simulink model "model_linear"  (R2022a)
settings: Solver=VariableStepAuto  StartTime=0  StopTime=100  RelTol=1e-3
values from neighbouring files (symbols this model uses):
  A = [ 0 1 0  0 ... (first row only)    [ball_and_beam_pfc.m]
  amplitude_entrada = 1    [ball_and_beam_pfc.m]
  B = [0 ... (first row only)    [ball_and_beam_pfc.m]
  bool_degrau = 1    [ball_and_beam_pfc.m]
  C = [0 0 1 0]    [ball_and_beam_pfc.m]
  k_seguimento = K_nulo(1:4)    [ball_and_beam_pfc.m]
  ki_seguimento = K_nulo(5)    [ball_and_beam_pfc.m]
  L = 0.425    [ball_and_beam_pfc.m]    (also in nonlinear_ball_and_beam.m)
libraries: vrlib x3
settings Model: Creator=Notebook_Artur  LastModifiedBy=Notebook_Artur

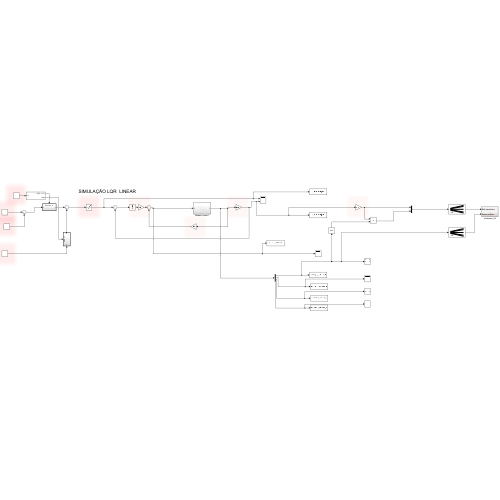
[thumbnail: Simulink's stored preview of the top-level diagram]
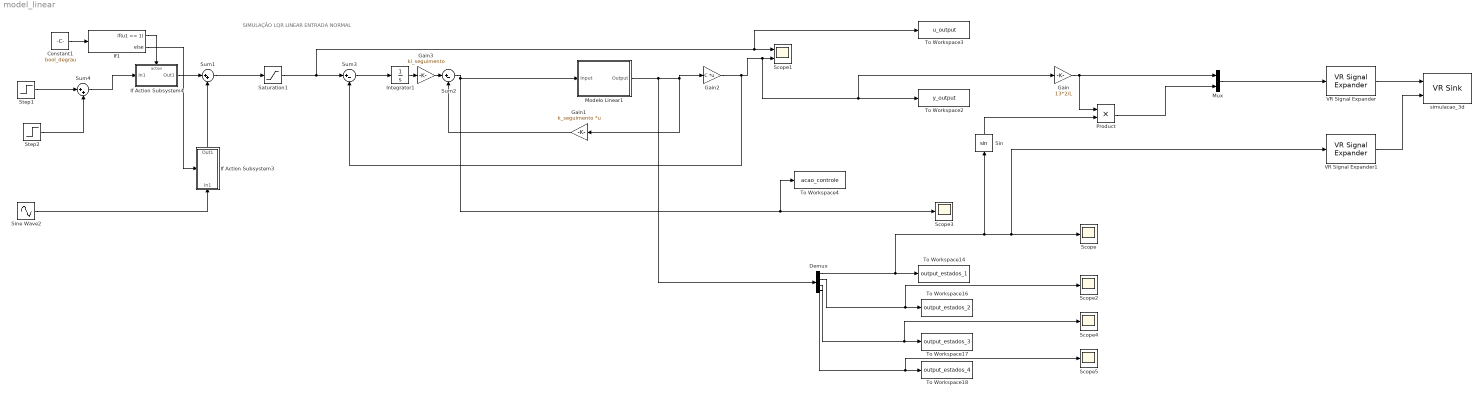
== system model_linear ==
  note: SIMULAÇÃO LQR LINEAR ENTRADA NORMAL
  Constant1 : Constant  Value=bool_degrau
  Demux : Demux
  Gain : Gain  Gain=13*2/L
  Gain1 : Gain  Gain=k_seguimento  Multiplication=Matrix(K*u)
  Gain2 : Gain  Gain=C  Multiplication=Matrix(K*u)
  Gain3 : Gain  Gain=ki_seguimento
  If Action Subsystem3 : Subsystem  TreatAsAtomicUnit=on
  If Action Subsystem4 : Subsystem  TreatAsAtomicUnit=on
  If1 : If  IfExpression=u1 == 1
  Integrator1 : Integrator
  Modelo Linear1 : Subsystem
  Mux : Mux  Inputs=2
  Product : Product
  Saturation1 : Saturate  UpperLimit=L/2  LowerLimit=-L/2
  Scope{,2..5} (5 alike) : Scope
  Scope1 : Scope  NumInputPorts=2
  Sin : Trigonometry
  Sine Wave2 : Sin  Amplitude=amplitude_entrada  Frequency=0.1  SampleTime=0
  Step1 : Step  After=amplitude_entrada  SampleTime=0
  Step2 : Step  Time=100  After=-2*amplitude_entrada  SampleTime=0
  Sum1 : Sum  Inputs=|++
  Sum2 : Sum  Inputs=|+-
  Sum3 : Sum  Inputs=|+-
  Sum4 : Sum  Inputs=|++
  To Workspace14 : ToWorkspace  VariableName=output_estados_1  SaveFormat=Timeseries  SampleTime=-1
  To Workspace16 : ToWorkspace  VariableName=output_estados_2  SaveFormat=Timeseries  SampleTime=-1
  To Workspace17 : ToWorkspace  VariableName=output_estados_3  SaveFormat=Timeseries  SampleTime=-1
  To Workspace18 : ToWorkspace  VariableName=output_estados_4  SaveFormat=Timeseries  SampleTime=-1
  To Workspace2 : ToWorkspace  VariableName=y_output  SaveFormat=Timeseries  SampleTime=-1
  To Workspace3 : ToWorkspace  VariableName=u_output  SaveFormat=Timeseries  SampleTime=-1
  To Workspace4 : ToWorkspace  VariableName=acao_controle  SaveFormat=Timeseries  SampleTime=-1
  VR Signal Expander : vrlib/VR Signal Expander  outwidth=3  outidx=[1 3]
  VR Signal Expander1 : vrlib/VR Signal Expander  outwidth=4  outidx=[4]
  simulacao_3d : vrlib/VR Sink  InstantiateOnLoad=on  SampleTime=0.1  ViewEnable=on  RemoteChange=off  RemoteView=off  FieldsWritten=Ball.translation.3.1.1.double#beam.rotation.4.1.1.double  WorldFileName=3d_ball_and_beam4.x3d  AutoView=on  VideoDimensions=[]  AllowVariableSize=off  FigureProperties="{'Position', 'Name', 'Viewpoint', 'CameraBound', 'CameraDirection', 'CameraPosition', 'CameraUpVector', 'ZoomFactor', 'Antialiasing', 'Headlight', 'Lighting', 'NavPanel', 'Sound', 'StatusBar', 'Stereo3D', 'Stereo3DCameraOffset', 'Stereo3DHIT', 'ToolBar', 'Textures', 'Transparency', 'Triad', 'Wireframe', 'NavZones', 'NavMode', 'NavSpeed', 'CaptureFileFormat', 'CaptureFileName', 'Record2DCompressMethod', 'Record2DCompressQuality', 'Record2D', 'Record2DFileName', 'Record2DFPS'; [5.0000000000000000e+00   9.2000000000000000e+01   5.7600000000000000e+02   3.5000000000000000e+02], '', '_untitled_1', 'on', [0.0000000000000000e+00   0.0000000000000000e+00  -1.0000000000000000e+00], [0.0000000000000000e+00   0.0000000000000000e+00   0.0000000000000000e+00], [0.0000000000000000e+00   1.0000000000000000e+00   0.0000000000000000e+00], [1.0000000000000000e+00], 'on', 'on', 'on', 'halfbar', 'on', 'on', 'off', [1.0000000149011612e-01], [0.0000000000000000e+00], 'on', 'on', 'on', 'none', 'off', 'off', 'fly', 'normal', 'tif', '%f_anim_%n.tif', 'auto', [7.5000000000000000e+01], 'off', '%f_anim_%n.avi', 'auto'}"
  wires:
  Sum4/1 -> If Action Subsystem4/1(In1)
  Demux/3 -> Scope4/1, To Workspace17/1
  Step2/1 -> Sum4/2
  Demux/4 -> Scope5/1, To Workspace18/1
  If Action Subsystem4/1(Out1) -> Sum1/1
  Demux/1 -> Scope/1, VR Signal Expander1/1, Sin/1, To Workspace14/1
  Modelo Linear1/1(Output) -> Demux/1, Gain2/1, Gain1/1
  If1/2 -> If Action Subsystem3/Action
  Demux/2 -> Scope2/1, To Workspace16/1
  If1/1 -> If Action Subsystem4/Action
  Sum2/1 -> Modelo Linear1/1(Input), Scope3/1, To Workspace4/1
  Gain2/1 -> Sum3/2, Gain/1, To Workspace2/1, Scope1/2
  Constant1/1 -> If1/1
  Step1/1 -> Sum4/1
  Integrator1/1 -> Gain3/1
  Gain1/1 -> Sum2/2
  Sum3/1 -> Integrator1/1
  Gain3/1 -> Sum2/1
  Saturation1/1 -> To Workspace3/1, Scope1/1, Sum3/1
  Sine Wave2/1 -> If Action Subsystem3/1(In1)
  If Action Subsystem3/1(Out1) -> Sum1/2
  VR Signal Expander/1 -> simulacao_3d/1
  VR Signal Expander1/1 -> simulacao_3d/2
  Sum1/1 -> Saturation1/1
  Mux/1 -> VR Signal Expander/1
  Gain/1 -> Product/1, Mux/1
  Sin/1 -> Product/2
  Product/1 -> Mux/2

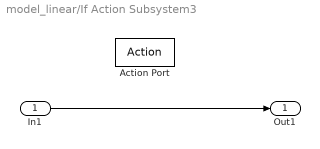
== system model_linear/If Action Subsystem3 ==
  In1 : Inport
  Action Port : ActionPort  ActionPortLabel=else
  Out1 : Outport
  wires:
  In1/1 -> Out1/1

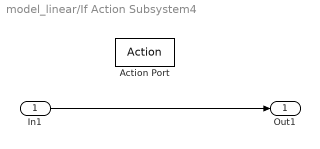
== system model_linear/If Action Subsystem4 ==
  In1 : Inport
  Action Port : ActionPort  ActionPortLabel=if(u1 == 1)
  Out1 : Outport
  wires:
  In1/1 -> Out1/1

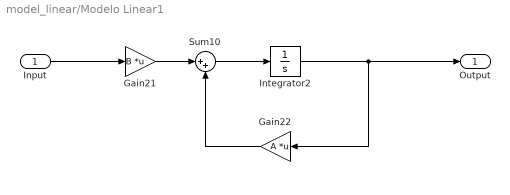
== system model_linear/Modelo Linear1 ==
  Input : Inport
  Gain21 : Gain  Gain=B  Multiplication=Matrix(K*u)
  Gain22 : Gain  Gain=A  Multiplication=Matrix(K*u)
  Integrator2 : Integrator
  Sum10 : Sum  Inputs=|++
  Output : Outport
  wires:
  Input/1 -> Gain21/1
  Gain22/1 -> Sum10/2
  Integrator2/1 -> Output/1, Gain22/1
  Gain21/1 -> Sum10/1
  Sum10/1 -> Integrator2/1
